simulink model "test_Wall_in"  (Simulink 7.6)
settings: Solver=ode23tb  StartTime=0.0  StopTime=100*24*3600  RelTol=1e-3
settings Model: Creator=drhf  LastModifiedBy=awohlfei
settings CodeAppCC: CustomSymbolStrType=$N$R$M_T

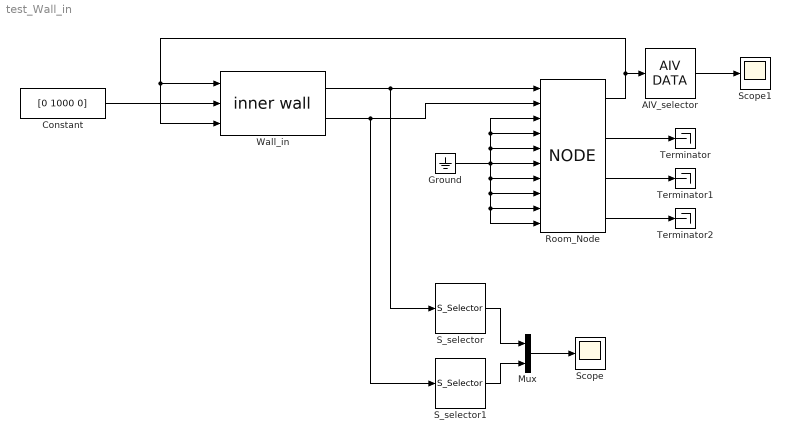
== system test_Wall_in ==
  AIV_selector : Reference  SystemSampleTime=-1  e1=on  e2=on  e3=on  e4=off  e5=off  e6=off  e7=off  e8=off  e9=off
  Constant : Constant  Value=[0 1000 0]
  Ground : Ground
  Mux : Mux  Inputs=2
  Room_Node : Reference  SystemSampleTime=-1  zoneairvolume=5*5*2.5  zoneheight=2.5  zonestartTEMP=20  zonestartWATER=55  timeconst=100  heatperfect=ideal profile (for heating demand)  lookuptime=[0 24]*3600  lookupvalue=[20 20]
  S_selector : Reference  SystemSampleTime=-1  e1=off  e2=off  e3=off  e4=off  e5=on  e6=off  e7=off  e8=off  e9=off  e10=off  e11=off  e12=off  e13=off
  S_selector1 : Reference  SystemSampleTime=-1  e1=off  e2=off  e3=off  e4=off  e5=on  e6=off  e7=off  e8=off  e9=off  e10=off  e11=off  e12=off  e13=off
  Scope : Scope
      settings: YMin=4  YMax=15
  Scope1 : Scope
      settings: SaveName=ScopeData2
  Terminator : Terminator
  Terminator1 : Terminator
  Terminator2 : Terminator
  Wall_in : Reference  SystemSampleTime=-1  wallsize=[10 10]  d=[0.1 0.1 0.1]  cond=[1 1 1]  cwall=[0.28 0.28 0.28]*3600  rho=[2000 200 2000]  emission_in=.96  t0=20  tau=1000*3600  dactive=[0.05 0.15 0.25]
  wires:
  Wall_in/1 -> Room_Node/1, S_selector/1
  Wall_in/2 -> Room_Node/2, S_selector1/1
  Ground/1 -> Room_Node/3, Room_Node/4, Room_Node/5, Room_Node/6, Room_Node/7, Room_Node/8, Room_Node/9, Room_Node/10
  Room_Node/1 -> Wall_in/1, Wall_in/3, AIV_selector/1
  Constant/1 -> Wall_in/2
  AIV_selector/1 -> Scope1/1
  Mux/1 -> Scope/1
  S_selector/1 -> Mux/1
  S_selector1/1 -> Mux/2
  Room_Node/2 -> Terminator/1
  Room_Node/3 -> Terminator1/1
  Room_Node/4 -> Terminator2/1
